simulink model "simu"  (R2015a)
settings: Solver=ode45  StartTime=0.0  StopTime=time  MaxStep=min([h hc ho])/50  RelTol=1e-5  AbsTol=1e-6
values from neighbouring files (symbols this model uses):
  A = [4,11,-30;1,0,0;0,1,0]    [main.m]
  Ad = zeros(size(A,1))    [main.m]
  AD = B*Kc/hc    [main.m]
  B = [1 1; 1 0; 0 1]    [main.m]
  C = eye(size(A,1))    [main.m]
  h = 0.2    [main.m]
  hc = 0.2    [main.m]
  ho = 0.2    [main.m]
  init = 10    [main.m]
  initialState = init*ones(size(A,1),1)*0.95    [main.m]
  K = place(A, B,[-2, -2.1, -2.2]*1.4)    [main.m]
  Ko = [5.65637568067253,9.81891791571489,-23.7635778046581 ... (first row only)    [main.m]
  L = place(A, B,[-2, -2.1, -2.2]*1.5)    [main.m]
  tn = max([h hc ho])    [main.m]
libraries: simulink x1
settings Model: Creator=matthieu  LastModifiedBy=matthieu

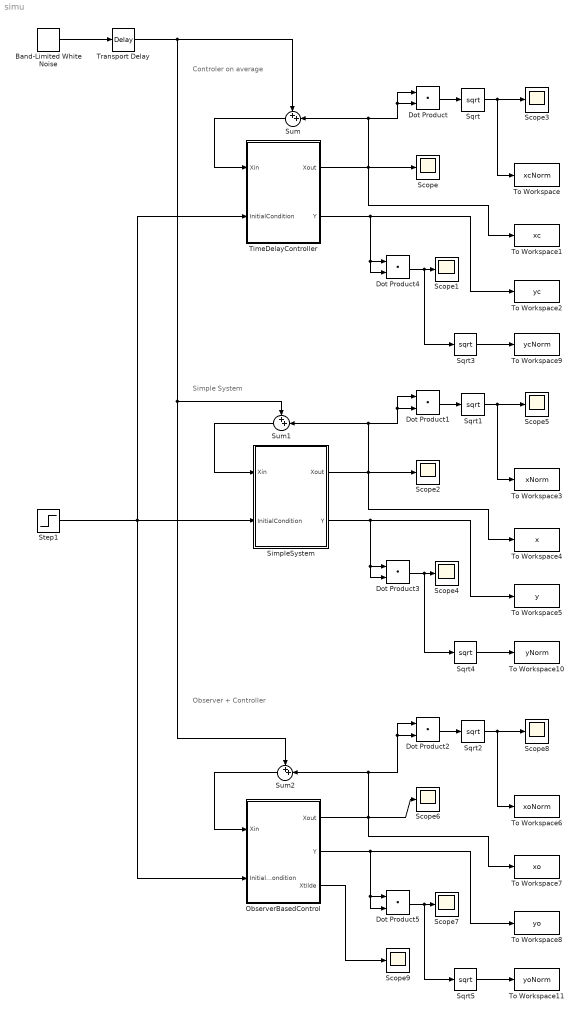
== system simu ==
  note: Observer + Controller
  note: Controler on average
  note: Simple System
  Band-Limited White Noise : simulink/Sources/Band-Limited White Noise  Cov=P  Ts=min([hc ho])/5  seed=[23341]
  Dot Product{,1..5} (6 alike) : DotProduct  InputSameDT=on  OutDataTypeStr=Inherit: Inherit via internal rule
  ObserverBasedControl : Subsystem
  Scope{,1..9} (10 alike) : Scope
      Scope settings: SaveName=ScopeData3
      Scope1 settings: SaveName=ScopeData4
      Scope2 settings: SaveName=ScopeData5
      Scope3 settings: SaveName=ScopeData6
      Scope4 settings: SaveName=ScopeData9
      Scope5 settings: SaveName=ScopeData10
      Scope6 settings: SaveName=ScopeData11
      Scope7 settings: SaveName=ScopeData12
      Scope8 settings: SaveName=ScopeData13
      Scope9 settings: SaveName=ScopeData16
  SimpleSystem : Subsystem
  Sqrt{,1..5} (6 alike) : Sqrt  SaturateOnIntegerOverflow=on
  Step1 : Step  Time=hc  Before=init*ones(size(A,1),1)  After=0  SampleTime=0
  Sum : Sum  Inputs=++|
  Sum1 : Sum  Inputs=++|
  Sum2 : Sum  Inputs=++|
  TimeDelayController : Subsystem
  To Workspace : ToWorkspace  VariableName=xcNorm  SaveFormat=Structure With Time  SampleTime=-1
      settings: Decimation=3
  To Workspace1 : ToWorkspace  VariableName=xc  SaveFormat=Structure With Time  SampleTime=-1
      settings: Decimation=3
  To Workspace10 : ToWorkspace  VariableName=yNorm  SaveFormat=Structure With Time  SampleTime=-1
      settings: Decimation=3
  To Workspace11 : ToWorkspace  VariableName=yoNorm  SaveFormat=Structure With Time  SampleTime=-1
      settings: Decimation=3
  To Workspace2 : ToWorkspace  VariableName=yc  SaveFormat=Structure With Time  SampleTime=-1
      settings: Decimation=3
  To Workspace3 : ToWorkspace  VariableName=xNorm  SaveFormat=Structure With Time  SampleTime=-1
      settings: Decimation=3
  To Workspace4 : ToWorkspace  VariableName=x  SaveFormat=Structure With Time  SampleTime=-1
      settings: Decimation=3
  To Workspace5 : ToWorkspace  VariableName=y  SaveFormat=Structure With Time  SampleTime=-1
      settings: Decimation=3
  To Workspace6 : ToWorkspace  VariableName=xoNorm  SaveFormat=Structure With Time  SampleTime=-1
      settings: Decimation=3
  To Workspace7 : ToWorkspace  VariableName=xo  SaveFormat=Structure With Time  SampleTime=-1
      settings: Decimation=3
  To Workspace8 : ToWorkspace  VariableName=yo  SaveFormat=Structure With Time  SampleTime=-1
      settings: Decimation=3
  To Workspace9 : ToWorkspace  VariableName=ycNorm  SaveFormat=Structure With Time  SampleTime=-1
      settings: Decimation=3
  Transport Delay : TransportDelay  DelayTime=tn
  wires:
  TimeDelayController/1(Xout) -> To Workspace1/1, Sum/2, Dot Product/1, Dot Product/2, Scope/1
  Dot Product/1 -> Sqrt/1
  Sqrt/1 -> To Workspace/1, Scope3/1
  Dot Product1/1 -> Sqrt1/1
  Sqrt1/1 -> To Workspace3/1, Scope5/1
  SimpleSystem/2(Y) -> Dot Product3/2, Dot Product3/1, To Workspace5/1
  Sum/1 -> TimeDelayController/1(Xin)
  SimpleSystem/1(Xout) -> To Workspace4/1, Dot Product1/1, Dot Product1/2, Sum1/2, Scope2/1
  Sum1/1 -> SimpleSystem/1(Xin)
  Dot Product2/1 -> Sqrt2/1
  Sqrt2/1 -> To Workspace6/1, Scope8/1
  Step1/1 -> TimeDelayController/2(InitialCondition), ObserverBasedControl/2(InitialCondition), SimpleSystem/2(InitialCondition)
  Band-Limited White Noise/1 -> Transport Delay/1
  ObserverBasedControl/1(Xout) -> Dot Product2/1, Dot Product2/2, Sum2/2, Scope6/1, To Workspace7/1
  Sum2/1 -> ObserverBasedControl/1(Xin)
  TimeDelayController/2(Y) -> Dot Product4/2, Dot Product4/1, To Workspace2/1
  Dot Product4/1 -> Sqrt3/1, Scope1/1
  ObserverBasedControl/2(Y) -> To Workspace8/1, Dot Product5/2, Dot Product5/1
  Sqrt3/1 -> To Workspace9/1
  Dot Product3/1 -> Sqrt4/1, Scope4/1
  Sqrt4/1 -> To Workspace10/1
  Dot Product5/1 -> Sqrt5/1, Scope7/1
  Sqrt5/1 -> To Workspace11/1
  Transport Delay/1 -> Sum2/1, Sum1/1, Sum/1
  ObserverBasedControl/3(Xtilde) -> Scope9/1

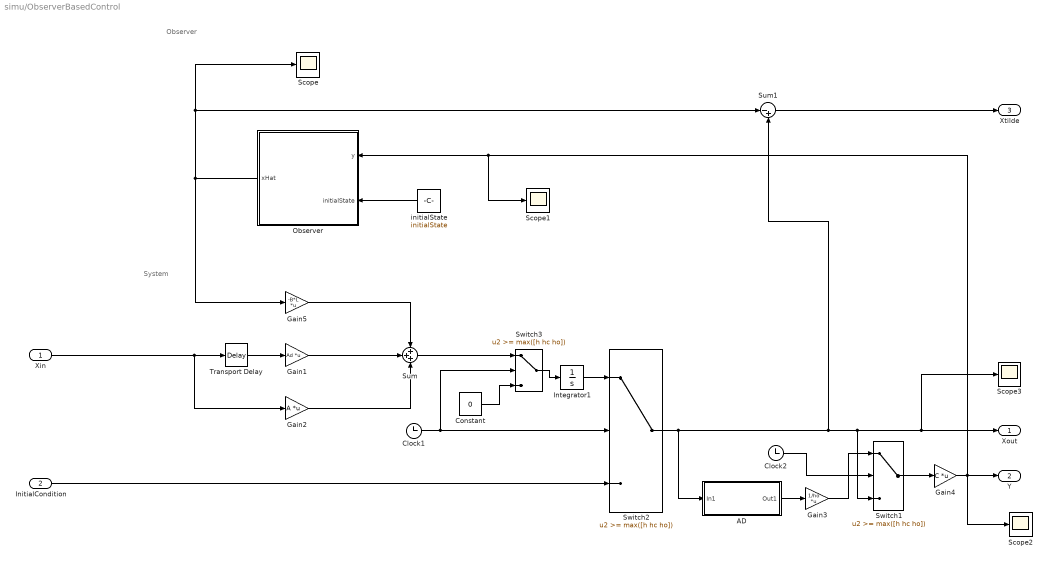
== system simu/ObserverBasedControl ==
  note: Observer
  note: System
  Xin : Inport
  InitialCondition : Inport  Port=2
  AD : Subsystem
  Clock1 : Clock
  Clock2 : Clock
  Constant : Constant  Value=0
  Gain1 : Gain  Gain=Ad  Multiplication=Matrix(K*u)
  Gain2 : Gain  Gain=A  Multiplication=Matrix(K*u)
  Gain3 : Gain  Gain=1/ho  Multiplication=Matrix(K*u)
  Gain4 : Gain  Gain=C  Multiplication=Matrix(K*u)
  Gain5 : Gain  Gain=-B*L  Multiplication=Matrix(K*u)
  Integrator1 : Integrator  InitialCondition=init*ones(size(A,1),1)
  Observer : Subsystem
  Scope{,1..3} (4 alike) : Scope
      Scope settings: TimeRange=5  SaveName=ScopeData14
      Scope1 settings: SaveName=ScopeData15
      Scope2 settings: SaveName=ScopeData17
      Scope3 settings: SaveName=ScopeData18
  Sum : Sum  Inputs=+++
  Sum1 : Sum  Inputs=|-+
  Switch1 : Switch  Threshold=max([h hc ho])  InputSameDT=on
      settings: LockScale=on
  Switch2 : Switch  Threshold=max([h hc ho])  InputSameDT=on
      settings: LockScale=on
  Switch3 : Switch  Threshold=max([h hc ho])  InputSameDT=on
      settings: LockScale=on
  Transport Delay : TransportDelay  DelayTime=ho
  initialState : Constant  Value=initialState
  Xout : Outport
  Y : Outport  Port=2
  Xtilde : Outport  Port=3
  wires:
  Transport Delay/1 -> Gain1/1
  Xin/1 -> Transport Delay/1, Gain2/1
  Gain2/1 -> Sum/3
  Clock1/1 -> Switch2/2, Switch3/2
  InitialCondition/1 -> Switch2/3
  Integrator1/1 -> Switch2/1
  Switch3/1 -> Integrator1/1
  Sum/1 -> Switch3/1
  Constant/1 -> Switch3/3
  Switch2/1 -> AD/1(In1), Switch1/3, Scope3/1, Xout/1, Sum1/2
  Gain1/1 -> Sum/2
  Gain5/1 -> Sum/1
  initialState/1 -> Observer/2(initialState)
  Observer/1(xHat) -> Scope/1, Sum1/1, Gain5/1
  Sum1/1 -> Xtilde/1
  AD/1(Out1) -> Gain3/1
  Switch1/1 -> Gain4/1
  Gain4/1 -> Scope2/1, Scope1/1, Observer/1(y), Y/1
  Gain3/1 -> Switch1/1
  Clock2/1 -> Switch1/2

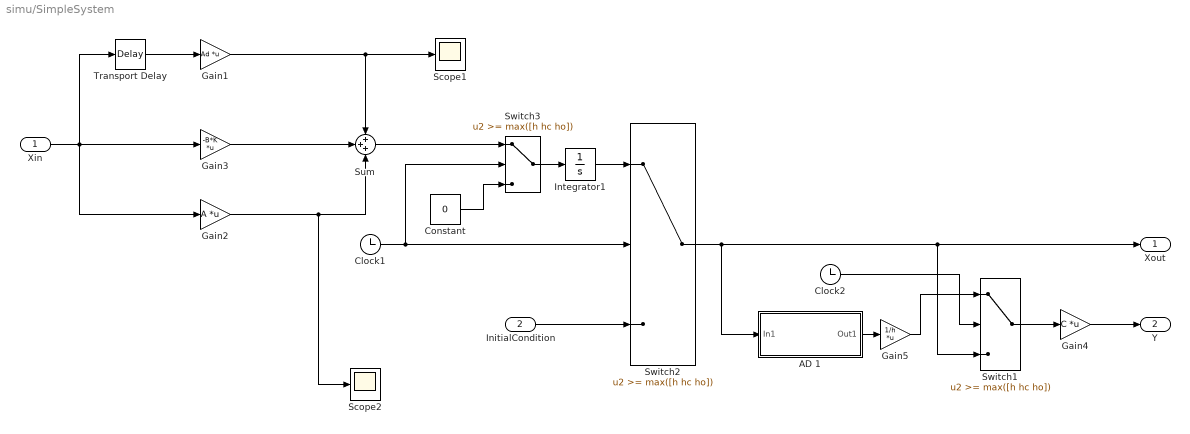
== system simu/SimpleSystem ==
  Xin : Inport
  InitialCondition : Inport  Port=2
  AD 1 : Subsystem
  Clock1 : Clock
  Clock2 : Clock
  Constant : Constant  Value=0
  Gain1 : Gain  Gain=Ad  Multiplication=Matrix(K*u)
  Gain2 : Gain  Gain=A  Multiplication=Matrix(K*u)
  Gain3 : Gain  Gain=-B*K  Multiplication=Matrix(K*u)
  Gain4 : Gain  Gain=C  Multiplication=Matrix(K*u)
  Gain5 : Gain  Gain=1/h  Multiplication=Matrix(K*u)
  Integrator1 : Integrator  InitialCondition=init*ones(size(A,1),1)
  Scope1 : Scope
      settings: SaveName=ScopeData7
  Scope2 : Scope
      settings: SaveName=ScopeData8
  Sum : Sum  Inputs=+++
  Switch1 : Switch  Threshold=max([h hc ho])  InputSameDT=on
      settings: LockScale=on
  Switch2 : Switch  Threshold=max([h hc ho])  InputSameDT=on
      settings: LockScale=on
  Switch3 : Switch  Threshold=max([h hc ho])  InputSameDT=on
      settings: LockScale=on
  Transport Delay : TransportDelay  DelayTime=h
  Xout : Outport
  Y : Outport  Port=2
  wires:
  Transport Delay/1 -> Gain1/1
  Gain1/1 -> Scope1/1, Sum/1
  Xin/1 -> Transport Delay/1, Gain3/1, Gain2/1
  Gain3/1 -> Sum/2
  Gain2/1 -> Scope2/1, Sum/3
  Clock1/1 -> Switch2/2, Switch3/2
  InitialCondition/1 -> Switch2/3
  Integrator1/1 -> Switch2/1
  Switch3/1 -> Integrator1/1
  Sum/1 -> Switch3/1
  Constant/1 -> Switch3/3
  Switch2/1 -> AD 1/1(In1), Switch1/3, Xout/1
  Gain4/1 -> Y/1
  AD 1/1(Out1) -> Gain5/1
  Clock2/1 -> Switch1/2
  Switch1/1 -> Gain4/1
  Gain5/1 -> Switch1/1

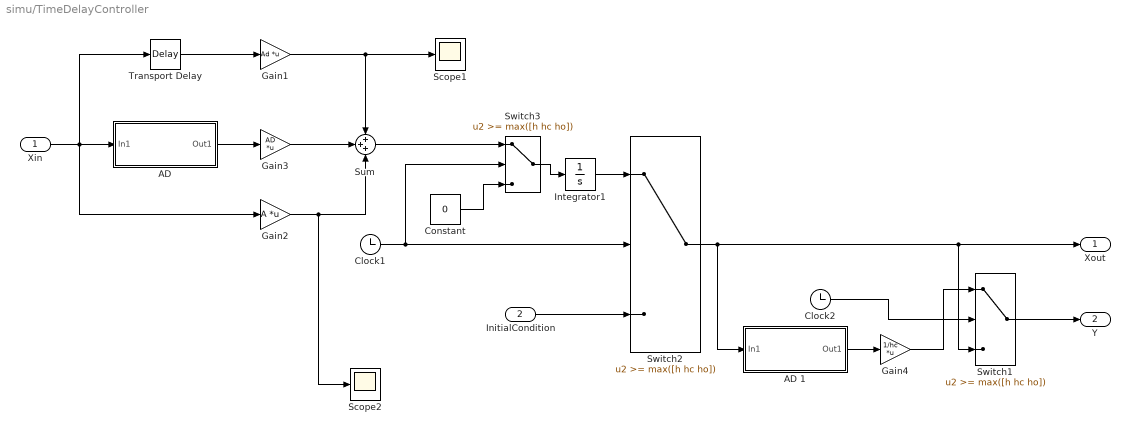
== system simu/TimeDelayController ==
  Xin : Inport
  InitialCondition : Inport  Port=2
  "AD " : Subsystem
  AD 1 : Subsystem
  Clock1 : Clock
  Clock2 : Clock
  Constant : Constant  Value=0
  Gain1 : Gain  Gain=Ad  Multiplication=Matrix(K*u)
  Gain2 : Gain  Gain=A  Multiplication=Matrix(K*u)
  Gain3 : Gain  Gain=AD  Multiplication=Matrix(K*u)
  Gain4 : Gain  Gain=1/hc  Multiplication=Matrix(K*u)
  Integrator1 : Integrator  InitialCondition=init*ones(size(A,1),1)
  Scope1 : Scope
      settings: SaveName=ScopeData7
  Scope2 : Scope
      settings: SaveName=ScopeData8
  Sum : Sum  Inputs=+++
  Switch1 : Switch  Threshold=max([h hc ho])  InputSameDT=on
      settings: LockScale=on
  Switch2 : Switch  Threshold=max([h hc ho])  InputSameDT=on
      settings: LockScale=on
  Switch3 : Switch  Threshold=max([h hc ho])  InputSameDT=on
      settings: LockScale=on
  Transport Delay : TransportDelay  DelayTime=hc
  Xout : Outport
  Y : Outport  Port=2
  wires:
  Transport Delay/1 -> Gain1/1
  Gain1/1 -> Scope1/1, Sum/1
  "AD "/1(Out1) -> Gain3/1
  Gain3/1 -> Sum/2
  Gain2/1 -> Scope2/1, Sum/3
  Xin/1 -> Gain2/1, Transport Delay/1, "AD "/1(In1)
  Clock1/1 -> Switch2/2, Switch3/2
  InitialCondition/1 -> Switch2/3
  Integrator1/1 -> Switch2/1
  Switch3/1 -> Integrator1/1
  Sum/1 -> Switch3/1
  Constant/1 -> Switch3/3
  Switch2/1 -> AD 1/1(In1), Switch1/3, Xout/1
  AD 1/1(Out1) -> Gain4/1
  Gain4/1 -> Switch1/1
  Clock2/1 -> Switch1/2
  Switch1/1 -> Y/1

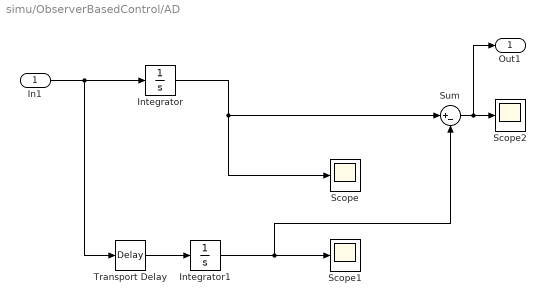
== system simu/ObserverBasedControl/AD ==
  In1 : Inport
  Integrator : Integrator
  Integrator1 : Integrator
  Scope : Scope
  Scope1 : Scope
  Scope2 : Scope
      settings: SaveName=ScopeData2
  Sum : Sum  Inputs=|+-
  Transport Delay : TransportDelay  DelayTime=ho
  Out1 : Outport
  wires:
  Sum/1 -> Scope2/1, Out1/1
  Integrator1/1 -> Scope1/1, Sum/2
  Transport Delay/1 -> Integrator1/1
  Integrator/1 -> Sum/1, Scope/1
  In1/1 -> Integrator/1, Transport Delay/1

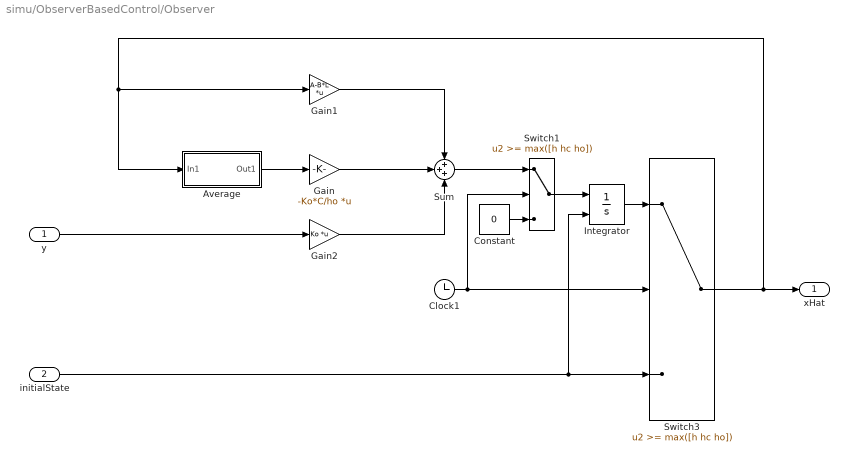
== system simu/ObserverBasedControl/Observer ==
  y : Inport
  initialState : Inport  Port=2
  Average : Subsystem
  Clock1 : Clock
  Constant : Constant  Value=0
  Gain : Gain  Gain=-Ko*C/ho  Multiplication=Matrix(K*u)
  Gain1 : Gain  Gain=A-B*L  Multiplication=Matrix(K*u)
  Gain2 : Gain  Gain=Ko  Multiplication=Matrix(K*u)
  Integrator : Integrator  InitialConditionSource=external
  Sum : Sum  Inputs=+++
  Switch1 : Switch  Threshold=max([h hc ho])  InputSameDT=on
      settings: LockScale=on
  Switch3 : Switch  Threshold=max([h hc ho])  InputSameDT=on
      settings: LockScale=on
  xHat : Outport
  wires:
  Average/1(Out1) -> Gain/1
  Gain/1 -> Sum/2
  Gain1/1 -> Sum/1
  Gain2/1 -> Sum/3
  y/1 -> Gain2/1
  initialState/1 -> Integrator/2, Switch3/3
  Integrator/1 -> Switch3/1
  Switch3/1 -> Gain1/1, Average/1(In1), xHat/1
  Clock1/1 -> Switch1/2, Switch3/2
  Switch1/1 -> Integrator/1
  Sum/1 -> Switch1/1
  Constant/1 -> Switch1/3

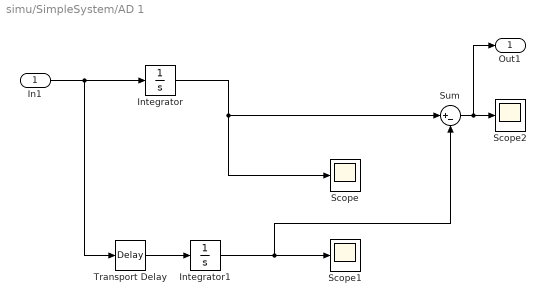
== system simu/SimpleSystem/AD 1 ==
  In1 : Inport
  Integrator : Integrator
  Integrator1 : Integrator
  Scope : Scope
  Scope1 : Scope
  Scope2 : Scope
      settings: SaveName=ScopeData2
  Sum : Sum  Inputs=|+-
  Transport Delay : TransportDelay  DelayTime=h
  Out1 : Outport
  wires:
  Sum/1 -> Scope2/1, Out1/1
  Integrator1/1 -> Scope1/1, Sum/2
  Transport Delay/1 -> Integrator1/1
  Integrator/1 -> Sum/1, Scope/1
  In1/1 -> Integrator/1, Transport Delay/1

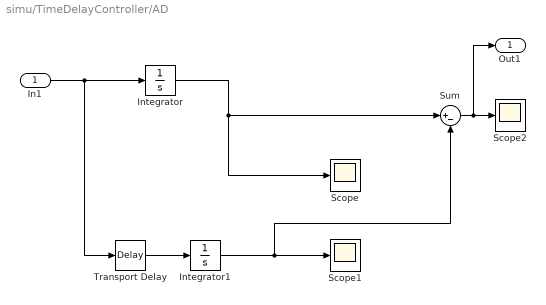
== system simu/TimeDelayController/AD  ==
  In1 : Inport
  Integrator : Integrator
  Integrator1 : Integrator
  Scope : Scope
  Scope1 : Scope
  Scope2 : Scope
      settings: SaveName=ScopeData2
  Sum : Sum  Inputs=|+-
  Transport Delay : TransportDelay  DelayTime=hc
  Out1 : Outport
  wires:
  In1/1 -> Transport Delay/1, Integrator/1
  Integrator/1 -> Scope/1, Sum/1
  Transport Delay/1 -> Integrator1/1
  Integrator1/1 -> Sum/2, Scope1/1
  Sum/1 -> Out1/1, Scope2/1

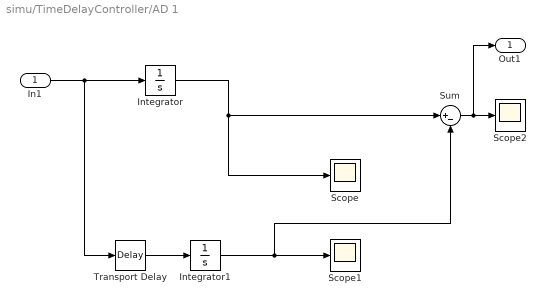
== system simu/TimeDelayController/AD 1 ==
  In1 : Inport
  Integrator : Integrator
  Integrator1 : Integrator
  Scope : Scope
  Scope1 : Scope
  Scope2 : Scope
      settings: SaveName=ScopeData2
  Sum : Sum  Inputs=|+-
  Transport Delay : TransportDelay  DelayTime=hc
  Out1 : Outport
  wires:
  Sum/1 -> Scope2/1, Out1/1
  Integrator1/1 -> Scope1/1, Sum/2
  Transport Delay/1 -> Integrator1/1
  Integrator/1 -> Sum/1, Scope/1
  In1/1 -> Integrator/1, Transport Delay/1

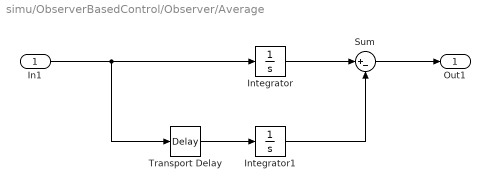
== system simu/ObserverBasedControl/Observer/Average ==
  In1 : Inport
  Integrator : Integrator
  Integrator1 : Integrator
  Sum : Sum  Inputs=|+-
  Transport Delay : TransportDelay  DelayTime=ho
  Out1 : Outport
  wires:
  Transport Delay/1 -> Integrator1/1
  Integrator1/1 -> Sum/2
  Integrator/1 -> Sum/1
  In1/1 -> Integrator/1, Transport Delay/1
  Sum/1 -> Out1/1
